simulink model "State_Calc"  (R2016b)
settings: Solver=FixedStepDiscrete  StartTime=0.0  StopTime=10  RelTol=1e-3
settings Model: Creator=3essawy  LastModifiedBy=3essawy
settings OptimizationCC: DefaultParameterBehavior=Inlined
settings DebuggingCC: ParameterTunabilityLossMsg=error
settings RTWCC: SystemTargetFile=ert.tlc  GenCodeOnly=on  TemplateMakefile=ert_default_tmf  Description=Embedded Coder  GenerateReport=on  IncludeHyperlinkInReport=on  LaunchReport=on  GenerateTraceInfo=on  GenerateTraceReport=on  GenerateTraceReportSl=on  GenerateTraceReportSf=on  GenerateTraceReportEml=on
settings CodeAppCC: ForceParamTrailComments=on  IgnoreCustomStorageClasses=off  OperatorAnnotations=on  SimulinkDataObjDesc=on  SFDataObjDesc=on  MATLABFcnDesc=on  InsertBlockDesc=on  MATLABSourceComments=on
settings ERTTargetCC: TargetLangStandard=C99 (ISO)  GenerateSampleERTMain=on  InlinedParameterPlacement=NonHierarchical  ERTCustomFileTemplate=example_file_process.tlc  EnableUserReplacementTypes=on

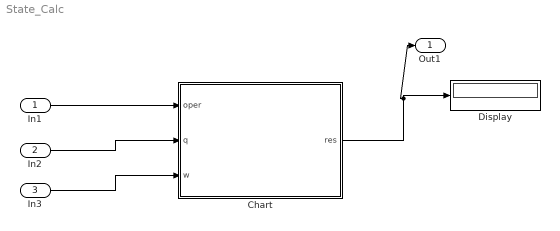
== system State_Calc ==
  In1 : Inport  OutDataTypeStr=uint8
  In2 : Inport  Port=2  OutDataTypeStr=uint8
  In3 : Inport  Port=3  OutDataTypeStr=uint8
  Chart : Stateflow chart  TreatAsAtomicUnit=on
  Display : Display
  Out1 : Outport
  wires:
  Chart/1(res) -> Out1/1, Display/1
  In1/1 -> Chart/1(oper)
  In3/1 -> Chart/3(w)
  In2/1 -> Chart/2(q)

== stateflow chart State_Calc/Chart ==
  state Calc(a, b, Operation) [function]
    note: Do not put any code along
        | the transitions that run
        | down the right side!
    (default) -> (junction 28)
    (junction 28) -> (junction 29) [order 1] : [Operation == 1]
    (junction 28) -> (junction 32) [order 2]
    (junction 29) -> (junction 30) : {res=a+b;}
    (junction 30) -> (junction 31)
    (junction 31) -> (junction 35)
    (junction 32) -> (junction 33) [order 1] : [Operation == 2]
    (junction 32) -> (junction 36) [order 2]
    (junction 33) -> (junction 34) : {res=a-b;}
    (junction 34) -> (junction 35)
    (junction 35) -> (junction 39)
    (junction 36) -> (junction 37) [order 1] : [Operation == 3]
    (junction 36) -> (junction 40) [order 2]
    (junction 37) -> (junction 38) : {res=a*b;}
    (junction 38) -> (junction 39)
    (junction 39) -> (junction 43)
    (junction 40) -> (junction 41) [order 1] : [Operation == 4]
    (junction 40) -> (junction 44) [order 2] : {res=a^b;}
    (junction 41) -> (junction 42) : {res=a/b;}
    (junction 42) -> (junction 43)
    (junction 43) -> (junction 45)
    (junction 45) -> (junction 44)
    (junction 44) -> (junction 46)
  (default) -> (junction 76) : {Calc(q,w,oper);}
  data: a function_input; b function_input; Operation function_input; oper input; q input; w input; res output
